simulink model "simpleio"  (Simulink 4.00)
settings: Solver=FixedStepDiscrete  StartTime=0.0  StopTime=10.0  RelTol=1e-3
libraries: intelligent x2
settings Model: Creator=quaranta  LastModifiedBy=quaranta  SaveTime=off  SaveOutput=off  SimulationMode=external  RTWOptions="-aExtMode=1 -aForceParamTrailComments=0 -aInlineInvariantSignals=0 -aInlineParameters=0 -aLocalBlockOutputs=1 -aLogVarNameModifier=\"rt_\" -aRTWVerbose=1 -aRollThreshold=5 -aShowEliminatedStatements=1"  RTWTemplateMakefile=grt_rtai.tmf  ExtModeTrigDuration=10000  BlockReductionOpt=off

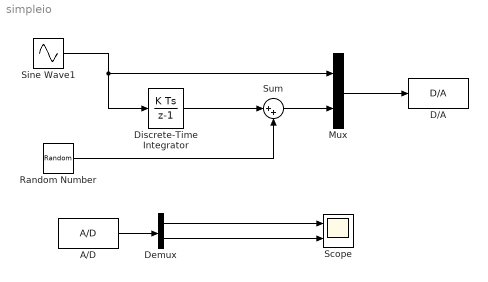
== system simpleio ==
  A/D : intelligent/A//D  AncestorBlock=mq3/A//D  n_ch=2  fs_ch=0  ts=1.e-4
  D/A : intelligent/D//A  AncestorBlock=mq3/D//A  n_ch=2  ts=1.e-4
  Demux : Demux  Outputs=2  BusSelectionMode=off
  Discrete-Time Integrator : DiscreteIntegrator  IntegratorMethod=ForwardEuler  ExternalReset=none  InitialConditionSource=internal  InitialCondition=0  LimitOutput=off  UpperSaturationLimit=inf  LowerSaturationLimit=-inf  ShowSaturationPort=off  ShowStatePort=off  SampleTime=1.e-4
  Mux : Mux  Inputs=2
  Random Number : RandomNumber  Mean=0  Variance=.5  Seed=0  SampleTime=1.e-4
  Scope : Scope  NumInputPorts=2
      settings: TimeRange=3  YMin=-5~-4.5  YMax=5~3  SaveToWorkspace=off  SaveName=ScopeData  MaxDataPoints=5000  Decimation=10
  Sine Wave1 : Sin  Amplitude=10  Frequency=10  Phase=0  SampleTime=1.e-4
  Sum : Sum  Inputs=|++  SaturateOnIntegerOverflow=on
  wires:
  Discrete-Time Integrator/1 -> Sum/1
  Random Number/1 -> Sum/2
  Sum/1 -> Mux/2
  Sine Wave1/1 -> Mux/1, Discrete-Time Integrator/1
  A/D/1 -> Demux/1
  Demux/1 -> Scope/1
  Demux/2 -> Scope/2
  Mux/1 -> D/A/1
